simulink model "Ozonation"  (Simulink 8.5)
settings: Solver=ode23tb  StartTime=0.0  StopTime=24*3600  MaxStep=1000  RelTol=1e-5  AbsTol=1e-5
undefined symbols (not defined in the file or in its folder): B, U, x0
settings Model: Creator=psross  LastModifiedBy=Martijn  ExtModeTrigMode=oneshot  ExtModeArmWhenConnect=off
settings DataIOCC: LimitDataPoints=off  SaveOutput=off  SaveTime=off  SignalLoggingName=sigsOut
settings OptimizationCC: BooleanDataType=off
settings DebuggingCC: SaveWithParameterizedLinksMsg=none  SignalResolutionControl=TryResolveAllWithWarning  MultiTaskDSMMsg=warning  MultiTaskCondExecSysMsg=none  FcnCallInpInsideContextMsg=UseLocalSettings  StrictBusMsg=None
settings HardwareCC: TargetUnknown=on

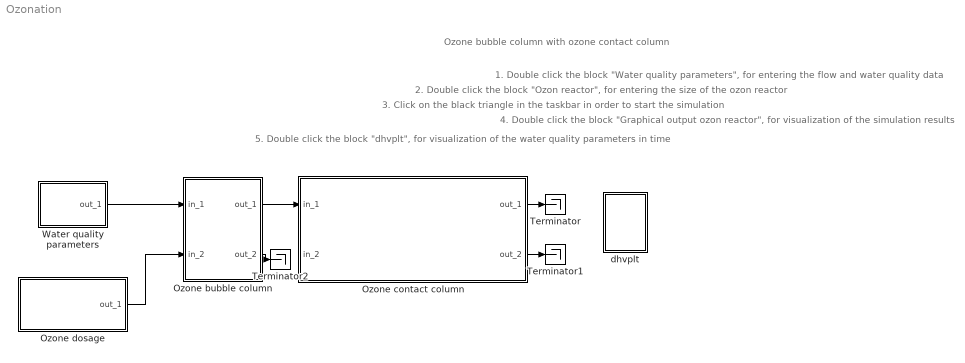
== system Ozonation ==
  note: 1. Double click the block "Water quality parameters", for entering the flow and water quality data
  note: 2. Double click the block "Ozon reactor", for entering the size of the ozon reactor
  note: 3. Click on the black triangle in the taskbar in order to start the simulation
  note: 4. Double click the block "Graphical output ozon reactor", for visualization of the simulation results
  note: Ozone bubble column with ozone contact column
  note: 5. Double click the block "dhvplt", for visualization of the water quality parameters in time
  Ozone bubble column : Subsystem
      mask init:
      | filenaam='./StimelaData/ozon_reactor_BC.mat';
      | 
      | [Pn,Fn,Fext]=Fileprop(filenaam);
      | 
      | errstr = st_UniqName(filenaam,'filenaam=''','SubSystem','OpenFcn');
      | if errstr, error([errstr 'The filename "' filenaam '" is already in use. Choose a different filename.']), end
      | 
      | P = ozonox_p(filenaam);
      | [B,x0,U]=ozonox_i(filenaam);
      settings: OpenFcn=|
      | filenaam='./StimelaData/ozon_reactor_BC.mat';
      | st_ParameterInput('init',gcb,filenaam,'ozonox');
      mask Display:
      | plot(0,0,100,100,[80,80,20,20],[80,20,20,80],[30,70,70,30,30],[31,31,29,29,31],[35,35],[38,35],[35,35],[48,45],[35,35],[58,55],[35,35],[68,65],[40,40],[41,38],[40,40],[51,48],[40,40],[61,58],[40,40],[71,68],[45,45],[34,31],[45,45],[44,41],[45,45],[54,51],[45,45],[64,61],[45,45],[74,71],[50,50],[38,35],[50,50],[48,45],[50,50],[58,55],[50,50],[68,65],[55,55],[41,38],[55,55],[51,48],[55,55],[61,58],[55,55],[71,68],[60,60],[34,31],[60,60],[44,41],[60,60],[54,51],[60,60],[64,61],[60,60],[74,71],[65,65],[38,35],[65,65],[48,45],[65,65],[58,55],[65,65],[68,65])
      | disp('')
      | text(50,50,'ozonox', 'horizontalAlignment', 'center', 'verticalAlignment', 'middle');
      | text(50,0,Fn, 'horizontalAlignment', 'center', 'verticalAlignment', 'base');
  Ozone contact column : Subsystem
      mask init:
      | filenaam='./StimelaData/ozon_reactor_CC.mat';
      | 
      | [Pn,Fn,Fext]=Fileprop(filenaam);
      | 
      | errstr = st_UniqName(filenaam,'filenaam=''','SubSystem','OpenFcn');
      | if errstr, error([errstr 'The filename "' filenaam '" is already in use. Choose a different filename.']), end
      | 
      | P = ozoncc_p(filenaam);
      | [B,x0,U]=ozoncc_i(filenaam);
      settings: OpenFcn=|
      | filenaam='./StimelaData/ozon_reactor_CC.mat';
      | st_ParameterInput('init',gcb,filenaam,'ozoncc');
      mask Display:
      | plot(0,0,100,100,[80,80,20,20],[80,20,20,80],[30,70,70,30,30],[31,31,29,29,31],[35,35],[38,35],[35,35],[48,45],[35,35],[58,55],[35,35],[68,65],[40,40],[41,38],[40,40],[51,48],[40,40],[61,58],[40,40],[71,68],[45,45],[34,31],[45,45],[44,41],[45,45],[54,51],[45,45],[64,61],[45,45],[74,71],[50,50],[38,35],[50,50],[48,45],[50,50],[58,55],[50,50],[68,65],[55,55],[41,38],[55,55],[51,48],[55,55],[61,58],[55,55],[71,68],[60,60],[34,31],[60,60],[44,41],[60,60],[54,51],[60,60],[64,61],[60,60],[74,71],[65,65],[38,35],[65,65],[48,45],[65,65],[58,55],[65,65],[68,65])
      | disp('')
      | text(50,50,'ozoncc', 'horizontalAlignment', 'center', 'verticalAlignment', 'middle');
      | text(50,0,Fn, 'horizontalAlignment', 'center', 'verticalAlignment', 'base');
  Ozone dosage : Subsystem  Description=ozodo1
      mask init:
      | filenaam='./StimelaData/ozon_reactor_OD.mat';
      | 
      | [Pn,Fn,Fext]=Fileprop(filenaam);
      | 
      | errstr = st_UniqName(filenaam,'filenaam=''','SubSystem','OpenFcn');
      | if errstr, error([errstr 'The filename "' filenaam '" is already in use. Choose a different filename.']), end
      | 
      | P = ozodo1_p(filenaam);
      | [B,x0,U]=ozodo1_i(filenaam);
      settings: OpenFcn=|
      | filenaam='./StimelaData/ozon_reactor_OD.mat';
      | st_ParameterInput('init',gcb,filenaam,'ozodo1');
      mask Display:
      | plot(0,0,100,100,[90,10],[10,10],[90,10],[30,30],[45,55,55,65,50,35,45,45],[90,90,50,50,30,50,50,90]);
      | disp('')
      | text(50,50,'ozodo1', 'horizontalAlignment', 'center', 'verticalAlignment', 'middle');
      | text(50,0,Fn, 'horizontalAlignment', 'center', 'verticalAlignment', 'base');
  Terminator : Terminator
  Terminator1 : Terminator
  Terminator2 : Terminator
  Water quality parameters : Subsystem  Description=The water flow and the water quality data must be filled out in the 'Water quality parameters' block. Each project must start with a 'Water quality parameters' block.
      mask init:
      | filenaam='./StimelaData/Water_qual_param.mat';
      | 
      | [Pn,Fn,Fext]=Fileprop(filenaam);
      | 
      | errstr = st_UniqName(filenaam,'filenaam=''','SubSystem','OpenFcn');
      | if errstr, error([errstr 'The filename "' filenaam '" is already in use. Choose a different filename.']), end
      | 
      | P = invruw_p(filenaam);
      | [B,x0,U]=invruw_i(filenaam);
      settings: OpenFcn=|
      | filenaam='./StimelaData/Water_qual_param.mat';
      | st_ParameterInput('init',gcb,filenaam,'invruw');
      mask Display:
      | plot(0,0,100,100,[80 100],[ 50 50],[80 100],[ 55 55],[20 80 80 20 20],[10 10 90  90 10]);
      | disp('')
      | text(50,50,'invruw', 'horizontalAlignment', 'center', 'verticalAlignment', 'middle');
      | text(50,0,Fn, 'horizontalAlignment', 'center', 'verticalAlignment', 'base');
  dhvplt : Subsystem
      settings: OpenFcn=plotStimela2
      mask Display:
      | plot(0,0,100,100,[80,20,20],[20,20,80],[80,69,60,52,45,39,33,28,24,20],[65,65,64,61,57,52,45,37,30,20])
      | disp('');
      | text(100,100,'Stimela', 'horizontalAlignment', 'right', 'verticalAlignment', 'top');
  wires:
  Water quality parameters/1(out_1) -> Ozone bubble column/1(in_1)
  Ozone dosage/1(out_1) -> Ozone bubble column/2(in_2)
  Ozone bubble column/1(out_1) -> Ozone contact column/1(in_1)
  Ozone contact column/1(out_1) -> Terminator/1
  Ozone contact column/2(out_2) -> Terminator1/1
  Ozone bubble column/2(out_2) -> Terminator2/1

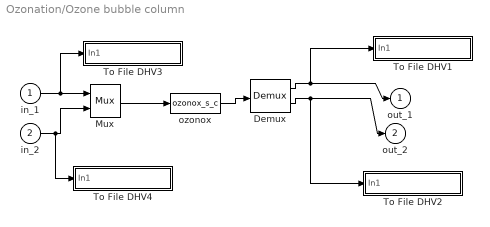
== system Ozonation/Ozone bubble column ==
  in_1 : Inport
  in_2 : Inport  Port=2
  Demux : Demux  Outputs=[U.Number B.Measurements]
  Mux : Mux  Inputs=[U.Number B.Setpoints]
  To File DHV1 : Subsystem  mask(To File DHV){naam=[filenaam(1:length(filenaam)-4) '_out.sti']}
      mask prompts: naam "Naam van bestand"
      mask init:
      | set_param([gcb '/To File'],'Filename',naam);
      mask Display: disp(naam)
  To File DHV2 : Subsystem  mask(To File DHV){naam=[filenaam(1:length(filenaam)-4) '_EM.sti']}
      mask prompts: naam "Naam van bestand"
      mask init:
      | set_param([gcb '/To File'],'Filename',naam);
      mask Display: disp(naam)
  To File DHV3 : Subsystem  mask(To File DHV){naam=[filenaam(1:length(filenaam)-4) '_in.sti']}
      mask prompts: naam "Naam van bestand"
      mask init:
      | set_param([gcb '/To File'],'Filename',naam);
      mask Display: disp(naam)
  To File DHV4 : Subsystem  mask(To File DHV){naam=[filenaam(1:length(filenaam)-4) '_ES.sti']}
      mask prompts: naam "Naam van bestand"
      mask init:
      | set_param([gcb '/To File'],'Filename',naam);
      mask Display: disp(naam)
  ozonox : S-Function  FunctionName=ozonox_s_c  Parameters=B,x0,U,P
  out_1 : Outport  InitialOutput=0
  out_2 : Outport  Port=2  InitialOutput=0
  wires:
  Demux/2 -> out_2/1, To File DHV2/1(In1)
  Demux/1 -> out_1/1, To File DHV1/1(In1)
  ozonox/1 -> Demux/1
  in_1/1 -> Mux/1, To File DHV3/1(In1)
  Mux/1 -> ozonox/1
  in_2/1 -> Mux/2, To File DHV4/1(In1)

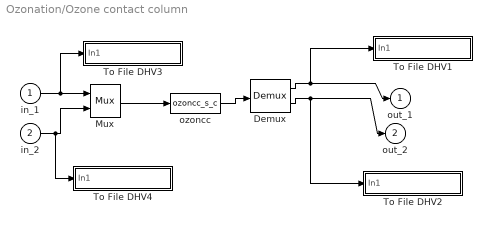
== system Ozonation/Ozone contact column ==
  in_1 : Inport
  in_2 : Inport  Port=2
  Demux : Demux  Outputs=[U.Number B.Measurements]
  Mux : Mux  Inputs=[U.Number B.Setpoints]
  To File DHV1 : Subsystem  mask(To File DHV){naam=[filenaam(1:length(filenaam)-4) '_out.sti']}
      mask prompts: naam "Naam van bestand"
      mask init:
      | set_param([gcb '/To File'],'Filename',naam);
      mask Display: disp(naam)
  To File DHV2 : Subsystem  mask(To File DHV){naam=[filenaam(1:length(filenaam)-4) '_EM.sti']}
      mask prompts: naam "Naam van bestand"
      mask init:
      | set_param([gcb '/To File'],'Filename',naam);
      mask Display: disp(naam)
  To File DHV3 : Subsystem  mask(To File DHV){naam=[filenaam(1:length(filenaam)-4) '_in.sti']}
      mask prompts: naam "Naam van bestand"
      mask init:
      | set_param([gcb '/To File'],'Filename',naam);
      mask Display: disp(naam)
  To File DHV4 : Subsystem  mask(To File DHV){naam=[filenaam(1:length(filenaam)-4) '_ES.sti']}
      mask prompts: naam "Naam van bestand"
      mask init:
      | set_param([gcb '/To File'],'Filename',naam);
      mask Display: disp(naam)
  ozoncc : S-Function  FunctionName=ozoncc_s_c  Parameters=B,x0,U,P
  out_1 : Outport  InitialOutput=0
  out_2 : Outport  Port=2  InitialOutput=0
  wires:
  Demux/2 -> out_2/1, To File DHV2/1(In1)
  Demux/1 -> out_1/1, To File DHV1/1(In1)
  ozoncc/1 -> Demux/1
  in_1/1 -> Mux/1, To File DHV3/1(In1)
  Mux/1 -> ozoncc/1
  in_2/1 -> Mux/2, To File DHV4/1(In1)

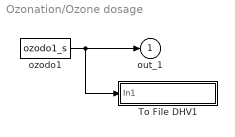
== system Ozonation/Ozone dosage ==
  To File DHV1 : Subsystem  mask(To File DHV){naam=[filenaam(1:length(filenaam)-4) '_out.sti']}
      mask prompts: naam "Naam van bestand"
      mask init:
      | set_param([gcb '/To File'],'Filename',naam);
      mask Display: disp(naam)
  ozodo1 : S-Function  FunctionName=ozodo1_s  Parameters=B,x0,U,P
  out_1 : Outport  InitialOutput=0
  wires:
  ozodo1/1 -> out_1/1, To File DHV1/1(In1)

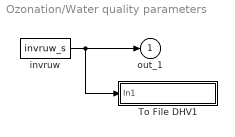
== system Ozonation/Water quality parameters ==
  To File DHV1 : Subsystem  mask(To File DHV){naam=[filenaam(1:length(filenaam)-4) '_out.sti']}
      mask prompts: naam "Naam van bestand"
      mask init:
      | set_param([gcb '/To File'],'Filename',naam);
      mask Display: disp(naam)
  invruw : S-Function  FunctionName=invruw_s  Parameters=B,x0,U,P
  out_1 : Outport  InitialOutput=0
  wires:
  invruw/1 -> out_1/1, To File DHV1/1(In1)

== system Ozonation/dhvplt ==
  note: plotten

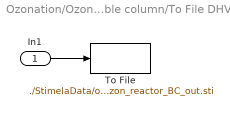
== system Ozonation/Ozone bubble column/To File DHV1 ==
  In1 : Inport
  To File : ToFile  Filename=./StimelaData/ozon_reactor_BC_out.sti  MatrixName=ozonoxout
  wires:
  In1/1 -> To File/1

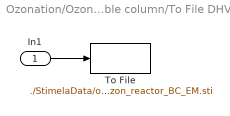
== system Ozonation/Ozone bubble column/To File DHV2 ==
  In1 : Inport
  To File : ToFile  Filename=./StimelaData/ozon_reactor_BC_EM.sti  MatrixName=ozonoxEM
  wires:
  In1/1 -> To File/1

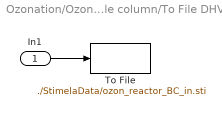
== system Ozonation/Ozone bubble column/To File DHV3 ==
  In1 : Inport
  To File : ToFile  Filename=./StimelaData/ozon_reactor_BC_in.sti  MatrixName=ozonoxin
  wires:
  In1/1 -> To File/1

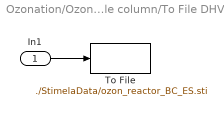
== system Ozonation/Ozone bubble column/To File DHV4 ==
  In1 : Inport
  To File : ToFile  Filename=./StimelaData/ozon_reactor_BC_ES.sti  MatrixName=ozonoxES
  wires:
  In1/1 -> To File/1

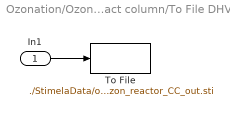
== system Ozonation/Ozone contact column/To File DHV1 ==
  In1 : Inport
  To File : ToFile  Filename=./StimelaData/ozon_reactor_CC_out.sti  MatrixName=ozonccout
  wires:
  In1/1 -> To File/1

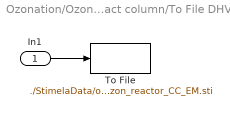
== system Ozonation/Ozone contact column/To File DHV2 ==
  In1 : Inport
  To File : ToFile  Filename=./StimelaData/ozon_reactor_CC_EM.sti  MatrixName=ozonccEM
  wires:
  In1/1 -> To File/1

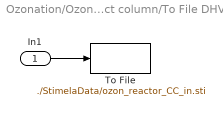
== system Ozonation/Ozone contact column/To File DHV3 ==
  In1 : Inport
  To File : ToFile  Filename=./StimelaData/ozon_reactor_CC_in.sti  MatrixName=ozonccin
  wires:
  In1/1 -> To File/1

== system Ozonation/Ozone contact column/To File DHV4 ==
  In1 : Inport
  To File : ToFile  Filename=./StimelaData/ozon_reactor_CC_ES.sti  MatrixName=ozonccES
  wires:
  In1/1 -> To File/1

== system Ozonation/Ozone dosage/To File DHV1 ==
  In1 : Inport
  To File : ToFile  Filename=./StimelaData/ozon_reactor_OD_out.sti  MatrixName=ozodo1out
  wires:
  In1/1 -> To File/1

== system Ozonation/Water quality parameters/To File DHV1 ==
  In1 : Inport
  To File : ToFile  Filename=./StimelaData/Water_qual_param_out.sti  MatrixName=invruwout
  wires:
  In1/1 -> To File/1
